simulink model "chaotic_descriptor"  (R2019b)
settings: Solver=VariableStepAuto  StartTime=0.0  StopTime=10.0  RelTol=1e-3
values from neighbouring files (symbols this model uses):
  x = fscanf(fileID, formatSpec)    [createDatabase.m]    (also in firstTest.m; lorenz.m = X(:,1))
undefined symbols (not defined in the file or in its folder): dim, tauOpt
settings Model: Creator=zuga_  LastModifiedBy=zuga_

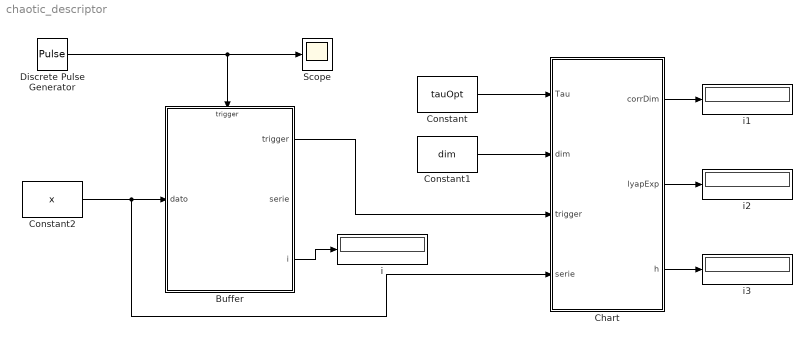
== system chaotic_descriptor ==
  Buffer : Stateflow chart  BlockKeywords=__PRM__SERIALIZED__DATA__:Stateflow Chart,Stateflow Diagram  TreatAsAtomicUnit=on
  Chart : Stateflow chart  BlockKeywords=__PRM__SERIALIZED__DATA__:Stateflow Chart,Stateflow Diagram  TreatAsAtomicUnit=on
  Constant : Constant  Value=tauOpt
  Constant1 : Constant  Value=dim
  Constant2 : Constant  Value=x
  Discrete Pulse Generator : DiscretePulseGenerator  PulseType=Time based  Period=1/173.62  PulseWidth=50
  Scope : Scope
  i{,1..3} (4 alike) : Display
  wires:
  Constant2/1 -> Chart/4(serie), Buffer/1(dato)
  Buffer/3(i) -> i/1
  Buffer/1(trigger) -> Chart/3(trigger)
  Discrete Pulse Generator/1 -> Scope/1, Buffer/Trigger
  Constant1/1 -> Chart/2(dim)
  Constant/1 -> Chart/1(Tau)
  Chart/3(h) -> i3/1
  Chart/2(lyapExp) -> i2/1
  Chart/1(corrDim) -> i1/1

== stateflow chart chaotic_descriptor/Buffer ==
  state AddData
    %en: serie = buffer(serie, i, dato);
    en: i = i+1;
  state Accelerate
    en: trigger = true;
  state End2
    en: trigger = false;
  (default) -> AddData : {
      | trigger = false;
      | size = 64;
      | serie = zeros(size, 1);
      | i = 1;
      | }
  AddData -> AddData [order 1] : [i < size]
  AddData -> Accelerate [order 2]
  Accelerate -> End2
  data: serie_in function_input; index function_input; data function_input; serie_out function_output; dato input double; trigger output boolean; serie output double size=5000; i output double; size local double
  events: event input RISING_EDGE_EVENT
  function serie_out = buffer(serie_in, index, data):
    | function serie_out = buffer(serie_in, index, data)
    |     if index == 1
    |         serie_out = data(((index-1)*64)+1:index*64-1);
    |     else
    |        serie_out = [serie_in data(((index-1)*64)+1:index*64-1)];
    |     end
    | end

== stateflow chart chaotic_descriptor/Chart ==
  (default) -> (junction 45)
  (junction 45) -> (junction 46) [order 1] : [trigger == true && flag == false]
  (junction 45) -> (junction 48) [order 2]
  (junction 46) -> (junction 47) : {
      | mean_period = meanperiod(serie, 173.61);
      | lyapExp = lyarosenstein(serie, Tau, 173.61, mean_period, 100);
      | corrDim = corrdim(serie, dim, Tau);
      | h = hurstexp(serie);
      | flag = true;
      | }
  (junction 47) -> (junction 48)
  (junction 48) -> (junction 56)
  data: x function_input; m function_input; tao function_input; npoint function_input; Y function_output; x function_input; Fs function_input; mp function_output; x function_input; m function_input; tau function_input; dg function_output; x function_input; m function_input; tao function_input; lle function_output; fs function_input; mean_period1 function_input; maxiter function_input; x function_input; H function_output; Tau input double size=1; dim input double size=1; trigger input boolean; serie input double; corrDim output double; lyapExp output double; h output double; flag local boolean; C_R local; R local; mean_period local
  function Y = psr_deneme(x,m,tao,npoint):
    | function Y = psr_deneme(x,m,tao,npoint)
    |   % Phase space reconstruction
    |   % x: time series
    |   % m: embedding dimension
    |   % tao: time delay
    |   % npoint: total number of reconstructed vectors
    |   % Y: M x m matrix
    |   % author: "MerveKizilkaya"
    | 
    |   N = length(x);
    |   if nargin == 4
    |     M = npoint;
    |   else
    |     M = N - (m-1)*tao;
    |   end
    |   Y = zeros(M, m);
    |   for i = 1:m
    |     Y(:, i) = x((1:M) + (i-1)*tao)';
    |   end
    | end
  function mp = meanperiod(x, Fs):
    | function mp = meanperiod(x, Fs)
    |   % Estimates the mean period of the time series
    |   % x: timeseries
    |   % Fs: samplingfrequency
    |   % Based upon the Matlab example obtained from:
    |   % http://www.mathworks.com/help/matlab/ref/fft.html
    |   % Band-Pass filter example was obtained from
    |   % http://www.mathworks.com/help/dsp/ref/fdesign.bandpass.html
    | 
    |   % T = 1/Fs;
    |   L = length(x);
    |   % t=(0:L - 1)*T;
    | 
    |   NFFT = 2^nextpow2(L); % Next power of 2 from length of y
    |   X = fft(x, NFFT)/L;
    |   f = Fs/2*linspace(0,1,NFFT/2 + 1);
    | 
    |   % % Plot single sided amplitude spectrum.
    |   figure
    |   plot(f, 2*abs(X(1:NFFT/2 + 1)))
    |   title('Single Sided Amplitude Spectrum of y(t)')
    |   xlabel('Frequency (Hz)')
    |   ylabel('|Y(f)|')
    |   mp = 1/(sum(2*abs(X(1:NFFT/2 + 1)))/length(X(1:NFFT/2 + 1)));
    | end
    | 
    | function y = butterworth(x)
    |   % Butterworth Filter for EEG time series
    |   fs = 173.61;
    | 
    |   %  Designan IIR Butterworth filter of order 10 with 3-dB
    |   %  frequencies of 0.53 and 60 Hz
    |   d = fdesign.bandpass('N,F3dB1,F3dB2', 10, 0.53, 60, fs);
    |   Hd = design(d,'butter');
    |   %  Apply the filter to the discrete-time signal.
    |   y = filter(Hd,x);
    |   figure(1)
    |   plot(x)
    |   xlabel('time');
    |   ylabel('microVolts');
    |   figure(2)
    |   plot(y)
    |   xlabel('time');
    |   ylabel('microVolts');
    |   xdft = fft(x);
    |   ydft = fft(y);
    |   % PlotResults
    |   freq = 0:(2*pi)/length(x):pi;
    |   plot(freq, abs(xdft(1:length(x)/2 + 1)));
    |   hold on;
    |   plot(freq, abs(ydft(1:length(x)/2 + 1)), 'r', 'linewidth', 2);
    |   legend('OriginalSignal', 'BandpassSignal');
    | end
  function dg = corrdim(x, m, tau):
    | function dg = corrdim(x, m, tau)
    |   % Correlation dimension based on Grassberger-Procaccia algorithm (1983)
    |   % dg: Correlation dimension
    |   % C_R: Vector of contribution of the points
    |   %     in the Radius R(size = (R_max - R_min/R_step) + 1)
    |   % R: Vector of radius(same size as C_R)
    |   % x: Time series
    |   % m: Embedded dimension
    |   % tau: Time delay
    |   % R_initial: Initial radius of the n-dimensional sphere (i.e. 0.3)
    |   % R_step: Increments of the radius(i.e. 0.1)
    |   % R_max: Max radius(-1 R_step) of the n-dimensional sphere
    |   %
    |   % Created by: Walther Carballo HernÃ¡ndez
    | 
    |   N = length(x);
    |   M = N - (m-1)*tau;
    |   % Attractor reconstruction
    |   Y = psr_deneme(x, m, tau);
    |   R_min = 1000;
    |   R_max = 0;
    |   % Distance vector between all the points size of N^2 - N
    |   dist_vec = zeros(1, ((N^2)-N));
    |   n = 1;
    |   % Estimating R_min and R_max
    |   for i=1:length(Y)                       % for each point
    |     for j=1:length(Y)                     % Compare with the other points
    |       if i~=j                             % if it's not the same point
    |       R_estimate = norm(Y(i,:)-Y(j,:));
    |       dist_vec(n) = R_estimate;
    |         if R_estimate<R_min               % Estimate min radius
    |           R_min = R_estimate;
    |         end
    |         if R_estimate>R_max               % Estimate max radius
    |           R_max = R_estimate;
    |         end
    |         n = n + 1;
    |       end
    |     end
    |   end
    |   % Range of the Radius ignore and 40% of the max radius
    |   R_range = 0.2*(R_max-R_min);
    |   R_max = R_max-2*R_range;
    |   if R_min == 0
    |     R_min = 1.0000e-06;% Solve some cases of NaN in R and C_R vectors
    |   end
    | 
    |   % Calculate step of the radius increase in the linear zone of 10 divisions
    |   R_step = (R_max-R_min)/10;
    |   R = R_min;
    |   C_R = zeros(1, floor(((R_max-R_min)/R_step) + 1));
    |   n = 1;
    |   sum = 0;
    | 
    |   % Obtaining C(R) vector
    |   while R <= R_max + 1                 % R_init tends to R_max in steps of R_step
    |     % for each distance in the distance vector
    |     for i=1:length(dist_vec)
    |       % if it's contained in the radius
    |       if dist_vec(i)<R
    |         % Add 1 to the counter
    |         sum = sum + 1;
    |       end
    |     end
    |     % C_R calculation
    |     C_R(n) = (2/(M*(M-1)))*sum;
    |     % Next step for the Radius
    |     R = R + R_step;
    |     sum = 0;
    |     n = n + 1;
    |   end
    |   % Calculate ln(C(R)) and ln(R)
    |   R = (R_min:R_step:R_max);
    |   lnC_R = log(C_R);
    |   lnR = log(R);
    |   % Calculate dg
    |   % coefficients = polyfit(lnR(2:length(lnR) - 5), lnC_R(2:length(lnC_R) - 5), 1);
    |   coefficients = polyfit(lnR(1:length(lnR) - 0), lnC_R(1:length(lnC_R) - 0), 1);
    |   % coefficients = polyfit(lnC_R(2:length(lnC_R) - 5), lnR(2:length(lnR) - 5), 1);
    |   % coefficients = polyfit(lnC_R(1:length(lnC_R) - 0), lnR(1:length(lnR) - 0), 1);
    |   % dg = 1/coefficients(1);
    |   dg = coefficients(1);
    |   % Plot results
    |   y = coefficients(1)*lnR + coefficients(2);
    |   figure
    |   hold on;
    |   plot(lnR, y, '--');
    |   plot(lnR, lnC_R);
    |   title('ln(C(R)) vs ln(R)');
    |   xlabel('ln(R)');
    |   ylabel('ln(C(R))');
    | end
  function lle = lyarosenstein(x,m,tao,fs,mean_period1,maxiter):
    | function lle = lyarosenstein(x,m,tao,fs,mean_period1,maxiter)
    |   % d: divergence of nearest trajectories
    |   % x: signal
    |   % tao: time delay
    |   % m: embedding dimension
    |   % fs: sampling frequency
    |   % Copyright(c) 2012, mirwais
    |   % All rights reserved.
    |   % Created by: Mirwais
    |   % Modifications by: Walther Carballo HernÃ¡ndez (2015)
    |   N = length(x);
    |   M = N-(m-1)*tao;
    |   Y = psr_deneme(x,m,tao);
    |   % Obtaining nearest distances
    |   for i=1:M
    |     x0 = ones(M,1)*Y(i,:);
    |     distance = sqrt(sum((Y-x0).^2,2));
    |     for j=1:M
    |       if abs(j-i)<=mean_period1
    |         distance(j) = 1e10;
    |       end
    |     end
    |     [neardis(i) nearpos(i)]=min(distance);
    |   end
    | 
    |   % Obtaining log of divergence
    |   for k=1:maxiter
    |     maxind = M-k;
    |     evolve = 0;
    |     pnt = 0;
    |     for j=1:M
    |       if j<= maxind && nearpos(j) <= maxind
    |         dist_k = sqrt(sum((Y(j + k, :) - Y(nearpos(j) + k, :)).^2, 2));
    |         if dist_k ~= 0
    |           evolve = evolve + log(dist_k);
    |           pnt = pnt + 1;
    |         end
    |       end
    |     end
    |     if pnt>0
    |       d(k) = evolve/pnt;
    |     else
    |       d(k) = 0;
    |     end
    |   end
    | 
    |   % figure
    |   % plot(d)
    | 
    | 
    |   % % LLE Calculation
    |   % tlinear = 1:1500;
    |   tlinear = 40:90;
    |   F = polyfit(tlinear,d(tlinear),1);
    |   lle = F(1)*fs;
    |   % Plot the results
    | 
    |   figure
    |   y = F(1)*d + F(2);
    |   % hold on
    |   % plot(d, y, '--')
    |   % plot(y)
    |   plot(d)
    |   title('Largest Lyapunov Exponent divergence');
    |   xlabel('Drive cycles');
    |   ylabel('LLE');
    | end
  function H=hurstexp(x):
    | function H=hurstexp(x)
    |   % Computing of Hurstexponent
    |   % x: time series
    |   % Created by: Walther Carballo HernÃ¡ndez
    | 
    |   % Length of the time series
    |   N = length(x);
    | 
    |   % Maximal 2-factors divisions of the time series
    |   max_divisions = round(log(N)/log(2));
    |   lnH_n = zeros(1, max_divisions);
    |   lnn = zeros(1, max_divisions);
    |   % for each division obtain the rescaled range
    |   for k=1:max_divisions
    |     n = round(N/(2^(k-1)));
    |     if (n==1)
    |       break;
    |     end
    |     lnn(k)=log(n);
    |     % Divide the time series
    |     X = x(1:n);
    |     % Obtaining the mean of the new time series
    |     m = mean(X);
    |     % Adjusting the time series to the mean
    |     Y = X-m;
    |     Z = zeros(1,n);
    |     R = 0;
    |     S = 0;
    |     sum = 0;
    |     % Computing the cumulative deviate series
    |     for t=1:n
    |       for i=1:t
    |         sum = sum + Y(i);
    |       end
    |       Z(t) = sum;
    |       sum = 0;
    |     end
    |     % Obtaining the range of the deviate series
    |     R = range(Z);
    |     % Computing standard deviation
    |     for i=1:n
    |       sum = sum + ((X(i)-m)^2);
    |     end
    |     S = sqrt((sum)/n);
    |     % Computing the results of rescaled range and store them
    |     if (isnan(log(R/S)))
    |       lnH_n(k) = 0;
    |     else
    |       lnH_n(k) = log(R/S);
    |     end
    |   end
    | 
    |   % Linear approximation
    |   coefficients = polyfit(lnn, lnH_n, 1);
    |   H = coefficients(1);
    |   % Plot results
    |   y = coefficients(1)*lnn + coefficients(2);
    |   figure;
    |   hold on;
    |   plot(lnn, y, '--');
    |   plot(lnn, lnH_n);
    |   title('ln(H(R/S)) vs ln(n)');
    |   xlabel('ln(n)');
    |   ylabel('ln(H(R/S))');
    | end
